simulink model "SimuOriginal"  (R2024b)
settings: Solver=ode4  StartTime=0.0  StopTime=180  FixedStep=Ts  RelTol=1e-3
values from neighbouring files (symbols this model uses):
  A_p = 4.2072e-4    (= 0.00042072)    [SI_NonLinear.m]
  A_t = pi*D_t^2/4    (= 1.25663706144e-05)    [SI_NonLinear.m]
  B_e = 3*10^-3    (= 0.003)    [SI_NonLinear.m]
  B_h = 0*17.26    (= 0)    [SI_NonLinear.m]
  b_v = 0.21    [SI_NonLinear.m]
  beta = 0.33*35    (= 11.55)    [SI_NonLinear.m]
  C_v = 4.5e-9    (= 4.5e-09)    [SI_NonLinear.m]
  D_t = 4e-3    (= 0.004)    [SI_NonLinear.m]
  K_e = 331    [SI_NonLinear.m]
  k_h = 0*243.2    (= 0)    [SI_NonLinear.m]
  K_v = 1/5    (= 0.2)    [SI_NonLinear.m]
  l_cyl = 0.275    [SI_NonLinear.m]
  L_t = 10    [SI_NonLinear.m]
  m_p = 0.25    [SI_NonLinear.m]
  mui = 1.813e-5    (= 1.813e-05)    [SI_NonLinear.m]
  omega_v = 150    [SI_NonLinear.m]
  P_atm = 1.013e5    (= 101300)    [SI_NonLinear.m]
  P_md = R*T*rho0    (= 101297.3962)    [SI_NonLinear.m]
  P_s = 3e5    (= 300000)    [SI_NonLinear.m]
  R = 287    [SI_NonLinear.m]
  rho0 = 1.204    [SI_NonLinear.m]
  T = 273.15+20    (= 293.15)    [SI_NonLinear.m]
  V_md = 2.4797*10^-5    (= 2.4797e-05)    [SI_NonLinear.m]
  V_sd = V_md    (= 2.4797e-05)    [SI_NonLinear.m]
  zeta_v = 0.7    [SI_NonLinear.m]
libraries: simulink x1
settings Model: Creator=user  LastModifiedBy=aha173
settings SolverCC: EnableFixedStepZeroCrossing=on

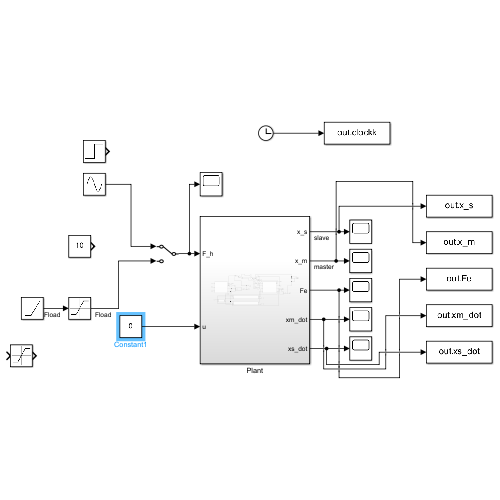
[thumbnail: Simulink's stored preview of the top-level diagram]
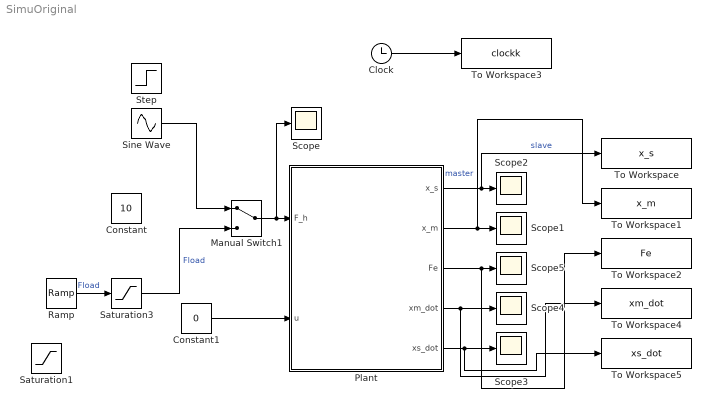
== system SimuOriginal ==
  Clock : Clock
  Constant : Constant  Value=10
  Constant1 : Constant  Value=0
  Manual Switch1 : ManualSwitch
  Plant : Subsystem
  Ramp : simulink/Sources/Ramp  slope=1  start=0  InitialOutput=0
  Saturation1 : Saturate  UpperLimit=10  LowerLimit=0
  Saturation3 : Saturate  UpperLimit=10  LowerLimit=0
  Scope{,1..5} (6 alike) : Scope
  Sine Wave : Sin  Amplitude=10  Bias=5  Frequency=0.5  SampleTime=0
  Step : Step  After=10  SampleTime=0
  To Workspace : ToWorkspace  VariableName=x_s  SaveFormat=Timeseries  SampleTime=-1
  To Workspace1 : ToWorkspace  VariableName=x_m  SaveFormat=Timeseries  SampleTime=-1
  To Workspace2 : ToWorkspace  VariableName=Fe  SaveFormat=Timeseries  SampleTime=-1
  To Workspace3 : ToWorkspace  VariableName=clockk  SampleTime=-1
  To Workspace4 : ToWorkspace  VariableName=xm_dot  SaveFormat=Timeseries  SampleTime=-1
  To Workspace5 : ToWorkspace  VariableName=xs_dot  SaveFormat=Timeseries  SampleTime=-1
  wires:
  Manual Switch1/1 -> Scope/1, Plant/1(F_h)
  Ramp/1 -> Saturation3/1  "Fload"
  Saturation3/1 -> Manual Switch1/2  "Fload"
  Sine Wave/1 -> Manual Switch1/1
  Clock/1 -> To Workspace3/1
  Plant/2(x_m) -> To Workspace1/1, Scope1/1  "master"
  Plant/1(x_s) -> To Workspace/1, Scope2/1  "slave"
  Plant/5(xs_dot) -> To Workspace5/1, Scope3/1
  Plant/4(xm_dot) -> To Workspace4/1, Scope4/1
  Plant/3(Fe) -> To Workspace2/1, Scope5/1
  Constant1/1 -> Plant/2(u)

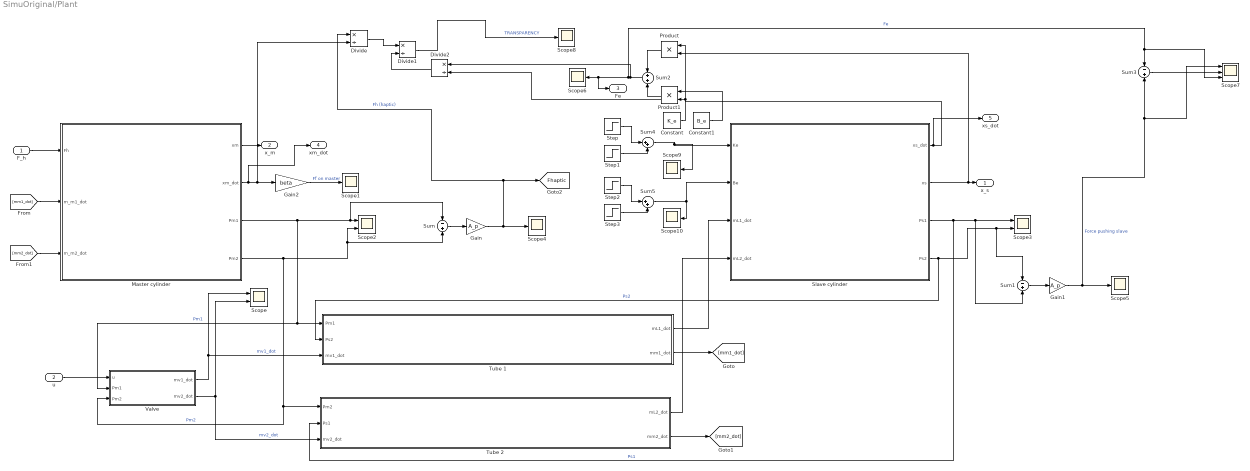
== system SimuOriginal/Plant ==
  F_h : Inport
  u : Inport  Port=2
  Constant : Constant  Value=K_e
  Constant1 : Constant  Value=B_e
  Divide : Product  Inputs=*/
  Divide1 : Product  Inputs=*/
  Divide2 : Product  Inputs=*/
  Gain : Gain  Gain=A_p
  Gain1 : Gain  Gain=A_p
  Gain2 : Gain  Gain=beta
  Master cylinder : Subsystem
  Product : Product
  Product1 : Product
  Scope : Scope  NumInputPorts=2
  Scope{1,4..6,8..10} (7 alike) : Scope
  Scope2 : Scope  NumInputPorts=2
  Scope3 : Scope  NumInputPorts=2
  Scope7 : Scope  NumInputPorts=3
  Slave cylinder : Subsystem
  Step : Step  Time=0  After=331  SampleTime=0
  Step1 : Step  Time=30  After=-248  SampleTime=0
  Step2 : Step  After=0.003  SampleTime=0
  Step3 : Step  Time=30  After=-0.002  SampleTime=0
  Sum : Sum  Inputs=-+
  Sum1 : Sum  Inputs=-+
  Sum2 : Sum
  Sum3 : Sum  Inputs=-+
  Sum4 : Sum  Inputs=|++
  Sum5 : Sum  Inputs=|++
  Tube 1 : Subsystem
  Tube 2 : Subsystem
  Valve : Subsystem
  x_s : Outport
  x_m : Outport  Port=2
  Fe : Outport  Port=3
  xm_dot : Outport  Port=4
  xs_dot : Outport  Port=5
  tag scope: Fhaptic=global
  wires:
  F_h/1 -> Master cylinder/1(Fh)
  u/1 -> Valve/1(u)
  Valve/1(mv1_dot) -> Tube 1/3(mv1_dot), Scope/1  "mv1_dot"
  Tube 1/2(mm1_dot) -> [mm1_dot]
  [mm1_dot] -> Master cylinder/2(m_m1_dot)
  Tube 2/2(mm2_dot) -> [mm2_dot]
  [mm2_dot] -> Master cylinder/3(m_m2_dot)
  Valve/2(mv2_dot) -> Scope/2, Tube 2/3(mv2_dot)  "mv2_dot"
  Constant1/1 -> Product1/1
  Slave cylinder/2(xs) -> Product/2, x_s/1
  Tube 1/1(mL1_dot) -> Slave cylinder/3(mL1_dot)
  Tube 2/1(mL2_dot) -> Slave cylinder/4(mL2_dot)
  Master cylinder/1(xm) -> x_m/1
  Master cylinder/3(Pm1) -> Sum/1, Scope2/1, Tube 1/1(Pm1), Valve/2(Pm1)  "Pm1"
  Master cylinder/4(Pm2) -> Scope2/2, Sum/2, Tube 2/1(Pm2), Valve/3(Pm2)  "Pm2"
  Sum/1 -> Gain/1
  Gain/1 -> Divide/1, [Fhaptic], Scope4/1  "Fh (haptic)"
  Gain1/1 -> Scope7/1, Sum3/2, Scope5/1  "Force pushing slave"
  Sum1/1 -> Gain1/1
  Master cylinder/2(xm_dot) -> xm_dot/1, Divide/2, Gain2/1
  Gain2/1 -> Scope1/1  "Ff on master"
  Product/1 -> Sum2/1
  Product1/1 -> Sum2/2
  Slave cylinder/1(xs_dot) -> xs_dot/1, Divide2/2, Product1/2
  Sum2/1 -> Fe/1, Scope6/1, Scope7/3, Sum3/1, Divide2/1  "Fe"
  Sum3/1 -> Scope7/2
  Slave cylinder/3(Ps1) -> Tube 2/2(Ps1), Sum1/2, Scope3/1  "Ps1"
  Slave cylinder/4(Ps2) -> Tube 1/2(Ps2), Sum1/1, Scope3/2  "Ps2"
  Divide/1 -> Divide1/1
  Divide2/1 -> Divide1/2
  Divide1/1 -> Scope8/1  "TRANSPARENCY"
  Step/1 -> Sum4/1
  Step1/1 -> Sum4/2
  Step2/1 -> Sum5/1
  Step3/1 -> Sum5/2
  Sum4/1 -> Scope9/1, Slave cylinder/1(Ke)
  Sum5/1 -> Scope10/1, Slave cylinder/2(Be)
  Constant/1 -> Product/1

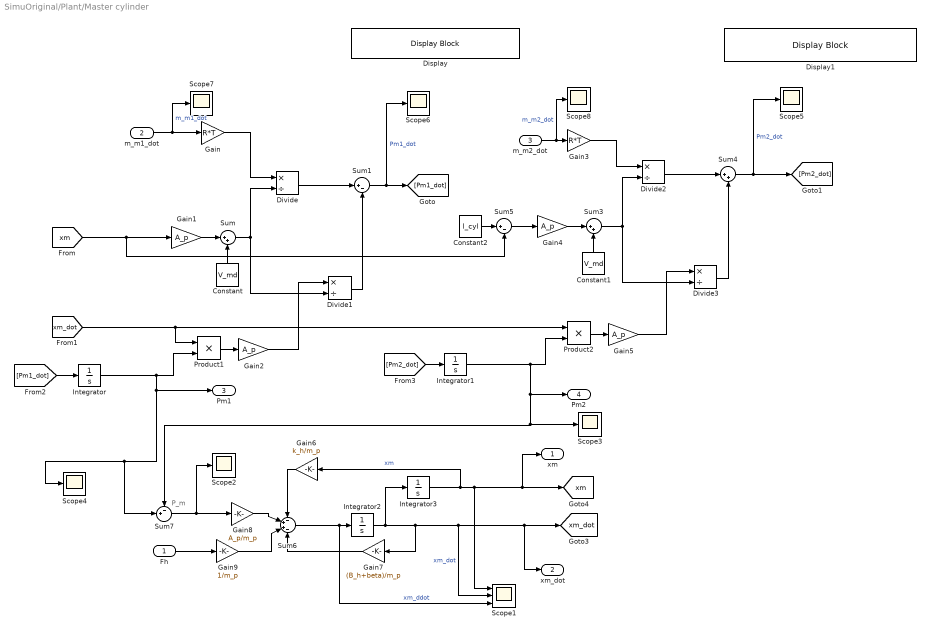
== system SimuOriginal/Plant/Master cylinder ==
  note: P_m
  Fh : Inport
  m_m1_dot : Inport  Port=2
  m_m2_dot : Inport  Port=3
  Constant : Constant  Value=V_md
  Constant1 : Constant  Value=V_md
  Constant2 : Constant  Value=l_cyl
  Display : DisplayBlock  LabelPosition=Hide  Format=long  Transparency=1
  Display1 : DisplayBlock  LabelPosition=Hide  Format=long  Transparency=1
  Divide{,1..3} (4 alike) : Product  Inputs=*/
  Gain : Gain  Gain=R*T
  Gain{1..2,4..5} (4 alike) : Gain  Gain=A_p
  Gain3 : Gain  Gain=R*T
  Gain6 : Gain  Gain=k_h/m_p
  Gain7 : Gain  Gain=(B_h+beta)/m_p
  Gain8 : Gain  Gain=A_p/m_p
  Gain9 : Gain  Gain=1/m_p
  Integrator : Integrator  InitialCondition=P_md
  Integrator1 : Integrator  InitialCondition=P_md
  Integrator2 : Integrator
  Integrator3 : Integrator
  Product1 : Product
  Product2 : Product
  Scope1 : Scope  NumInputPorts=3
  Scope{2..8} (7 alike) : Scope
  Sum : Sum  Inputs=|++
  Sum1 : Sum  Inputs=|+-
  Sum3 : Sum  Inputs=|++
  Sum4 : Sum  Inputs=|++
  Sum5 : Sum  Inputs=|+-
  Sum6 : Sum  Inputs=-++-
  Sum7 : Sum  Inputs=-+|
  xm : Outport
  xm_dot : Outport  Port=2
  Pm1 : Outport  Port=3
  Pm2 : Outport  Port=4
  tag scope: xm=global, xm_dot=global
  wires:
  Constant/1 -> Sum/2
  Gain1/1 -> Sum/1
  Gain/1 -> Divide/1
  m_m1_dot/1 -> Scope7/1, Gain/1  "m_m1_dot"
  Sum/1 -> Divide1/2, Divide/2
  Product1/1 -> Gain2/1
  Gain2/1 -> Divide1/1
  Divide/1 -> Sum1/1
  Divide1/1 -> Sum1/2
  m_m2_dot/1 -> Scope8/1, Gain3/1  "m_m2_dot"
  Gain3/1 -> Divide2/1
  Sum3/1 -> Divide3/2, Divide2/2
  Gain4/1 -> Sum3/1
  Gain5/1 -> Divide3/1
  Constant1/1 -> Sum3/2
  Product2/1 -> Gain5/1
  [xm_dot] -> Product1/1, Product2/1
  Divide2/1 -> Sum4/1
  Divide3/1 -> Sum4/2
  Sum5/1 -> Gain4/1
  [xm] -> Sum5/2, Gain1/1
  Constant2/1 -> Sum5/1
  Sum1/1 -> Scope6/1, [Pm1_dot]  "Pm1_dot"
  Sum4/1 -> Scope5/1, [Pm2_dot]  "Pm2_dot"
  Integrator3/1 -> xm/1, [xm], Scope1/1, Gain6/1  "xm"
  Gain7/1 -> Sum6/4
  Sum6/1 -> Scope1/3, Integrator2/1  "xm_ddot"
  Fh/1 -> Gain9/1
  Sum7/1 -> Gain8/1, Scope2/1
  Gain6/1 -> Sum6/1
  Gain9/1 -> Sum6/3
  Integrator2/1 -> Integrator3/1, Scope1/2, xm_dot/1, [xm_dot], Gain7/1  "xm_dot"
  [Pm1_dot] -> Integrator/1
  [Pm2_dot] -> Integrator1/1
  Gain8/1 -> Sum6/2
  Integrator/1 -> Pm1/1, Scope4/1, Sum7/2, Product1/2
  Integrator1/1 -> Pm2/1, Sum7/1, Scope3/1, Product2/2

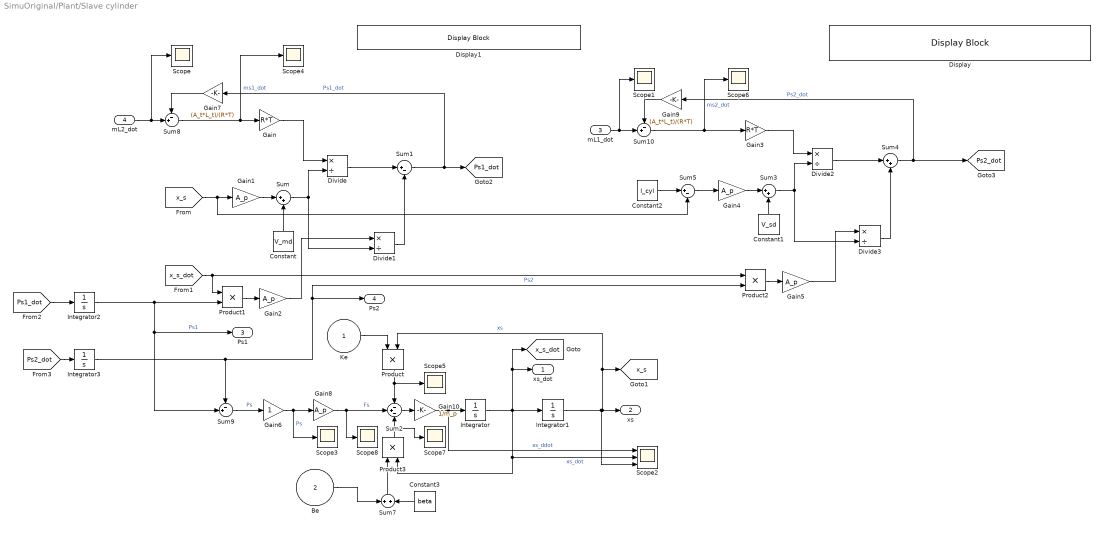
== system SimuOriginal/Plant/Slave cylinder ==
  Ke : Inport
  Be : Inport  Port=2
  mL1_dot : Inport  Port=3
  mL2_dot : Inport  Port=4
  Constant : Constant  Value=V_md
  Constant1 : Constant  Value=V_sd
  Constant2 : Constant  Value=l_cyl
  Constant3 : Constant  Value=beta
  Display : DisplayBlock  LabelPosition=Hide  Format=long  Transparency=1
  Display1 : DisplayBlock  LabelPosition=Hide  Format=long  Transparency=1
  Divide{,1..3} (4 alike) : Product  Inputs=*/
  Gain : Gain  Gain=R*T
  Gain{1..2,4..5,8} (5 alike) : Gain  Gain=A_p
  Gain10 : Gain  Gain=1/m_p
  Gain3 : Gain  Gain=R*T
  Gain6 : Gain
  Gain7 : Gain  Gain=(A_t*L_t)/(R*T)
  Gain9 : Gain  Gain=(A_t*L_t)/(R*T)
  Integrator : Integrator
  Integrator1 : Integrator
  Integrator2 : Integrator  InitialCondition=P_md
  Integrator3 : Integrator  InitialCondition=P_md
  Product{,1..3} (4 alike) : Product
  Scope{,1,3..8} (8 alike) : Scope
  Scope2 : Scope  NumInputPorts=3
  Sum : Sum  Inputs=|++
  Sum1 : Sum  Inputs=|+-
  Sum10 : Sum  Inputs=-+|
  Sum2 : Sum  Inputs=-+-
  Sum3 : Sum  Inputs=|++
  Sum4 : Sum  Inputs=|++
  Sum5 : Sum  Inputs=|+-
  Sum7 : Sum
  Sum8 : Sum  Inputs=-+|
  Sum9 : Sum  Inputs=-+|
  xs_dot : Outport
  xs : Outport  Port=2
  Ps1 : Outport  Port=3
  Ps2 : Outport  Port=4
  tag scope: Ps1_dot=global, Ps2_dot=global, x_s=global, x_s_dot=global
  wires:
  Sum4/1 -> Gain9/1, [Ps2_dot]  "Ps2_dot"
  Sum1/1 -> Gain7/1, [Ps1_dot]  "Ps1_dot"
  Divide2/1 -> Sum4/1
  Sum10/1 -> Scope6/1, Gain3/1  "ms2_dot"
  Gain4/1 -> Sum3/1
  Sum5/1 -> Gain4/1
  Divide3/1 -> Sum4/2
  Gain5/1 -> Divide3/1
  Constant2/1 -> Sum5/1
  Product1/1 -> Gain2/1
  Product2/1 -> Gain5/1
  Sum/1 -> Divide1/2, Divide/2
  Sum3/1 -> Divide3/2, Divide2/2
  Divide/1 -> Sum1/1
  Gain3/1 -> Divide2/1
  Divide1/1 -> Sum1/2
  Constant1/1 -> Sum3/2
  Gain/1 -> Divide/1
  Constant/1 -> Sum/2
  Gain2/1 -> Divide1/1
  Gain1/1 -> Sum/1
  Product/1 -> Scope5/1, Sum2/1
  Ke/1 -> Product/1
  Sum9/1 -> Gain6/1  "Ps"
  Integrator1/1 -> Scope2/3, Product/2, [x_s], xs/1  "xs"
  Gain8/1 -> Sum2/2, Scope8/1  "Fs"
  Sum2/1 -> Gain10/1
  [x_s] -> Sum5/2, Gain1/1
  mL2_dot/1 -> Scope/1, Sum8/2
  Gain7/1 -> Sum8/1
  Sum8/1 -> Scope4/1, Gain/1  "ms1_dot"
  [x_s_dot] -> Product2/1, Product1/1
  mL1_dot/1 -> Scope1/1, Sum10/2
  Gain9/1 -> Sum10/1
  Gain10/1 -> Scope2/1, Integrator/1  "xs_ddot"
  [Ps1_dot] -> Integrator2/1
  Integrator2/1 -> Ps1/1, Sum9/2, Product1/2  "Ps1"
  [Ps2_dot] -> Integrator3/1
  Integrator3/1 -> Product2/2, Ps2/1, Sum9/1  "Ps2"
  Product3/1 -> Scope7/1, Sum2/3
  Be/1 -> Sum7/1
  Constant3/1 -> Sum7/2
  Sum7/1 -> Product3/1
  Integrator/1 -> Product3/2, Scope2/2, Integrator1/1, [x_s_dot], xs_dot/1  "xs_dot"
  Gain6/1 -> Gain8/1, Scope3/1  "Ps"

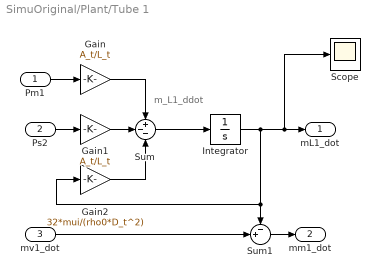
== system SimuOriginal/Plant/Tube 1 ==
  note: m_L1_ddot
  Pm1 : Inport
  Ps2 : Inport  Port=2
  mv1_dot : Inport  Port=3
  Gain : Gain  Gain=A_t/L_t
  Gain1 : Gain  Gain=A_t/L_t
  Gain2 : Gain  Gain=32*mui/(rho0*D_t^2)
  Integrator : Integrator
  Scope : Scope
  Sum : Sum  Inputs=+--
  Sum1 : Sum  Inputs=-+|
  mL1_dot : Outport
  mm1_dot : Outport  Port=2
  wires:
  Pm1/1 -> Gain/1
  Gain/1 -> Sum/1
  Integrator/1 -> Scope/1, mL1_dot/1, Sum1/1, Gain2/1
  Gain1/1 -> Sum/2
  Ps2/1 -> Gain1/1
  Gain2/1 -> Sum/3
  Sum/1 -> Integrator/1
  Sum1/1 -> mm1_dot/1
  mv1_dot/1 -> Sum1/2

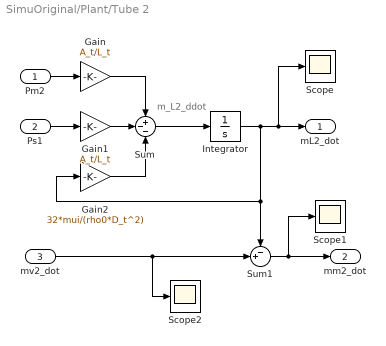
== system SimuOriginal/Plant/Tube 2 ==
  note: m_L2_ddot
  Pm2 : Inport
  Ps1 : Inport  Port=2
  mv2_dot : Inport  Port=3
  Gain : Gain  Gain=A_t/L_t
  Gain1 : Gain  Gain=A_t/L_t
  Gain2 : Gain  Gain=32*mui/(rho0*D_t^2)
  Integrator : Integrator
  Scope : Scope
  Scope1 : Scope
  Scope2 : Scope
  Sum : Sum  Inputs=+--
  Sum1 : Sum  Inputs=-+|
  mL2_dot : Outport
  mm2_dot : Outport  Port=2
  wires:
  Pm2/1 -> Gain/1
  Gain/1 -> Sum/1
  Integrator/1 -> Scope/1, mL2_dot/1, Sum1/1, Gain2/1
  Gain1/1 -> Sum/2
  Ps1/1 -> Gain1/1
  Gain2/1 -> Sum/3
  Sum/1 -> Integrator/1
  Sum1/1 -> Scope1/1, mm2_dot/1
  mv2_dot/1 -> Scope2/1, Sum1/2

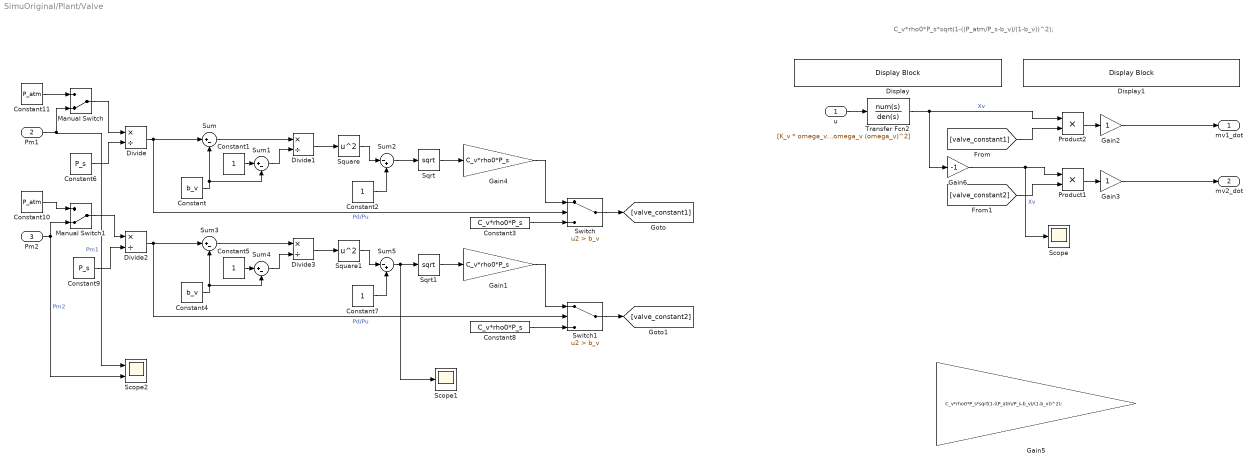
== system SimuOriginal/Plant/Valve ==
  note: C_v*rho0*P_s*sqrt(1-((P_atm/P_s-b_v)/(1-b_v))^2);
  u : Inport
  Pm1 : Inport  Port=2
  Pm2 : Inport  Port=3
  Constant : Constant  Value=b_v
  Constant{1..2,5,7} (4 alike) : Constant
  Constant10 : Constant  Value=P_atm
  Constant11 : Constant  Value=P_atm
  Constant3 : Constant  Value=C_v*rho0*P_s
  Constant4 : Constant  Value=b_v
  Constant6 : Constant  Value=P_s
  Constant8 : Constant  Value=C_v*rho0*P_s
  Constant9 : Constant  Value=P_s
  Display : DisplayBlock  Format=long  Transparency=1
  Display1 : DisplayBlock  Format=long  Transparency=1
  Divide{,1..3} (4 alike) : Product  Inputs=*/
  Gain1 : Gain  Gain=C_v*rho0*P_s
  Gain2 : Gain
  Gain3 : Gain
  Gain4 : Gain  Gain=C_v*rho0*P_s
  Gain5 : Gain  Gain=C_v*rho0*P_s*sqrt(1-((P_atm/P_s-b_v)/(1-b_v))^2);
  Gain6 : Gain  Gain=-1
  Manual Switch : ManualSwitch  CurrentSetting=0
  Manual Switch1 : ManualSwitch  CurrentSetting=0
  Product1 : Product
  Product2 : Product
  Scope : Scope
  Scope1 : Scope
  Scope2 : Scope  NumInputPorts=2
  Sqrt : Sqrt
  Sqrt1 : Sqrt
  Square : Math  Operator=square
  Square1 : Math  Operator=square
  Sum{,1,3..4} (4 alike) : Sum  Inputs=|+-
  Sum2 : Sum  Inputs=|-+
  Sum5 : Sum  Inputs=|-+
  Switch : Switch  Criteria=u2 > Threshold  Threshold=b_v  SaturateOnIntegerOverflow=off  InputSameDT=off
  Switch1 : Switch  Criteria=u2 > Threshold  Threshold=b_v  SaturateOnIntegerOverflow=off  InputSameDT=off
  Transfer Fcn2 : TransferFcn  Numerator=[K_v * omega_v^2]  Denominator=[1 2*zeta_v*omega_v (omega_v)^2]
  mv1_dot : Outport
  mv2_dot : Outport  Port=2
  wires:
  Divide/1 -> Switch/2, Sum/1  "Pd/Pu"
  Constant/1 -> Sum1/2, Sum/2
  Sum/1 -> Divide1/1
  Sum1/1 -> Divide1/2
  Constant1/1 -> Sum1/1
  Divide1/1 -> Square/1
  Square/1 -> Sum2/1
  Constant2/1 -> Sum2/2
  Sum2/1 -> Sqrt/1
  Sqrt/1 -> Gain4/1
  [valve_constant1] -> Product2/2
  Constant6/1 -> Divide/2
  Gain4/1 -> Switch/1
  Constant3/1 -> Switch/3
  Switch/1 -> [valve_constant1]
  Product2/1 -> Gain2/1
  Gain1/1 -> Switch1/1
  Constant8/1 -> Switch1/3
  Switch1/1 -> [valve_constant2]
  Constant5/1 -> Sum4/1
  Constant4/1 -> Sum4/2, Sum3/2
  Divide3/1 -> Square1/1
  Square1/1 -> Sum5/1
  Sum3/1 -> Divide3/1
  Constant7/1 -> Sum5/2
  Sum4/1 -> Divide3/2
  Sqrt1/1 -> Gain1/1
  Divide2/1 -> Switch1/2, Sum3/1  "Pd/Pu"
  Sum5/1 -> Scope1/1, Sqrt1/1
  [valve_constant2] -> Product1/2
  Constant9/1 -> Divide2/2
  Product1/1 -> Gain3/1
  u/1 -> Transfer Fcn2/1
  Gain6/1 -> Scope/1, Product1/1  "Xv"
  Pm1/1 -> Scope2/1, Manual Switch/2  "Pm1"
  Constant11/1 -> Manual Switch/1
  Manual Switch/1 -> Divide/1
  Constant10/1 -> Manual Switch1/1
  Pm2/1 -> Scope2/2, Manual Switch1/2  "Pm2"
  Manual Switch1/1 -> Divide2/1
  Transfer Fcn2/1 -> Gain6/1, Product2/1  "Xv"
  Gain2/1 -> mv1_dot/1
  Gain3/1 -> mv2_dot/1
